simulink model "WFXXPIDzlsa"  (Simulink 5.0)
settings: Solver=ode4  SolverMode=SingleTasking  StartTime=0.0  StopTime=8000  FixedStep=10  RelTol=1e-3
settings Model: LastModifiedBy=ThinkPad

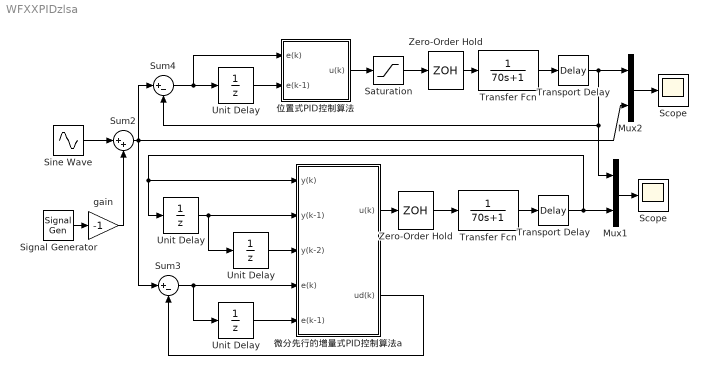
== system WFXXPIDzlsa ==
  " Unit Delay " : UnitDelay  SampleTime=20
  Mux1 : Mux  Inputs=2
  Mux2 : Mux  Inputs=2
  Saturation : Saturate  UpperLimit=10  LowerLimit=-10
  Scope : Scope
      settings: YMin=-1.5  YMax=1.5  SaveName=Scope10  DataFormat=Array  MaxDataPoints=500000
  "Scope " : Scope
      settings: YMin=-3.5  YMax=1  SaveName=ScopeData3  MaxDataPoints=500000
  Signal Generator : SignalGenerator  WaveForm=square  Frequency=0.0005*pi  Units=rad/sec
  Sine Wave : Sin  Amplitude=0.05  Frequency=0.03*pi  SampleTime=0
  Sum2 : Sum  Inputs=|++  SaturateOnIntegerOverflow=on
  Sum3 : Sum  Inputs=|+-  SaturateOnIntegerOverflow=on
  Sum4 : Sum  Inputs=|+-  SaturateOnIntegerOverflow=on
  Transfer Fcn : TransferFcn  Denominator=[70 1]
  "Transfer Fcn " : TransferFcn  Denominator=[70 1]
  Transport Delay : TransportDelay  DelayTime=80
  "Transport Delay " : TransportDelay  DelayTime=80
  Unit Delay : UnitDelay  SampleTime=20
  "Unit Delay " : UnitDelay  SampleTime=20
  "Unit Delay  " : UnitDelay  SampleTime=20
  Zero-Order Hold : ZeroOrderHold  SampleTime=20
  "Zero-Order Hold " : ZeroOrderHold  SampleTime=20
  gain : Gain  Gain=-1  SaturateOnIntegerOverflow=on
  微分先行的增量式PID控制算法a : Subsystem
  "位置式PID控制算法 " : Subsystem
  wires:
  Sum2/1 -> Sum4/1, Mux2/2, Sum3/1
  Transfer Fcn/1 -> Transport Delay/1
  "位置式PID控制算法 "/1(u(k)) -> Saturation/1
  Sum4/1 -> Unit Delay/1, "位置式PID控制算法 "/1(e(k))
  Zero-Order Hold/1 -> Transfer Fcn/1
  Mux2/1 -> Scope/1
  Transport Delay/1 -> Mux2/1, Sum4/2, Mux1/1
  Unit Delay/1 -> "位置式PID控制算法 "/2(e(k-1))
  Sine Wave/1 -> Sum2/1
  Signal Generator/1 -> gain/1
  gain/1 -> Sum2/2
  Saturation/1 -> Zero-Order Hold/1
  Sum3/1 -> 微分先行的增量式PID控制算法a/4(e(k)), "Unit Delay  "/1
  Mux1/1 -> "Scope "/1
  "Transport Delay "/1 -> "Unit Delay "/1, 微分先行的增量式PID控制算法a/1(y(k)), Mux1/2
  微分先行的增量式PID控制算法a/1(u(k)) -> "Zero-Order Hold "/1
  "Unit Delay "/1 -> " Unit Delay "/1, 微分先行的增量式PID控制算法a/2(y(k-1))
  "Unit Delay  "/1 -> 微分先行的增量式PID控制算法a/5(e(k-1))
  " Unit Delay "/1 -> 微分先行的增量式PID控制算法a/3(y(k-2))
  "Transfer Fcn "/1 -> "Transport Delay "/1
  "Zero-Order Hold "/1 -> "Transfer Fcn "/1
  微分先行的增量式PID控制算法a/2(ud(k)) -> Sum3/2

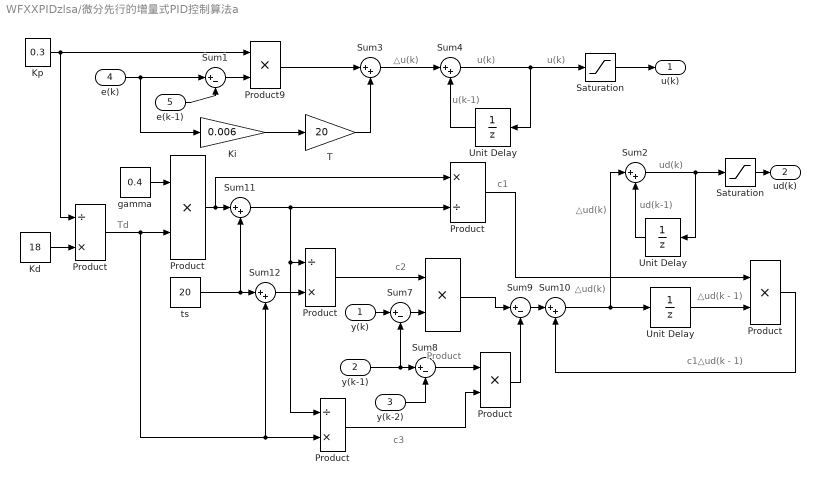
== system WFXXPIDzlsa/微分先行的增量式PID控制算法a ==
  note: u(k-1)
  note: △u(k)
  note: u(k)
  note: c1△ud(k－1)
  note: Td
  note: c2
  note: c3
  note: c1
  note: u(k)
  note: △ud(k－1)
  note: △ud(k)
  note: ud(k-1)
  note: △ud(k)
  note: ud(k)
  note: Product
  y(k) : Inport
  y(k-1) : Inport  Port=2
  y(k-2) : Inport  Port=3
  e(k) : Inport  Port=4
  e(k-1) : Inport  Port=5
  " " : Product  SaturateOnIntegerOverflow=on
  "   Product " : Product  SaturateOnIntegerOverflow=on
  "  Product " : Product  Inputs=/*  SaturateOnIntegerOverflow=on
  "  Product  " : Product  Inputs=/*  SaturateOnIntegerOverflow=on
  "  Product   " : Product  Inputs=/*  SaturateOnIntegerOverflow=on
  " Product " : Product  Inputs=*/  SaturateOnIntegerOverflow=on
  Kd : Constant  Value=18
  Ki : Gain  Gain=0.006  SaturateOnIntegerOverflow=on
  Kp : Constant  Value=0.3
  Product : Product  SaturateOnIntegerOverflow=on
  "Product  " : Product  SaturateOnIntegerOverflow=on
  Product9 : Product  SaturateOnIntegerOverflow=on
  Saturation : Saturate  UpperLimit=10  LowerLimit=-10
  "Saturation " : Saturate  UpperLimit=10  LowerLimit=-10
  Sum{1,7..9} (4 alike) : Sum  Inputs=|+-  SaturateOnIntegerOverflow=on
  Sum{2..4,10..12} (6 alike) : Sum  Inputs=|++  SaturateOnIntegerOverflow=on
  T : Gain  Gain=20  SaturateOnIntegerOverflow=on
  Unit Delay : UnitDelay  Orientation=left  SampleTime=20
  "Unit Delay " : UnitDelay  SampleTime=20
  "Unit Delay  " : UnitDelay  Orientation=left  SampleTime=20
  gamma : Constant  Value=0.4
  ts : Constant  Value=20
  u(k) : Outport
  ud(k) : Outport  Port=2
  wires:
  Product9/1 -> Sum3/1
  Ki/1 -> T/1
  Sum4/1 -> Unit Delay/1, Saturation/1
  Unit Delay/1 -> Sum4/2
  e(k-1)/1 -> Sum1/2
  Sum3/1 -> Sum4/1
  Product/1 -> Sum10/2
  Sum9/1 -> Sum10/1
  Sum10/1 -> "Unit Delay "/1, Sum2/1
  Kp/1 -> "  Product   "/1, Product9/1
  Kd/1 -> "  Product   "/2
  "Product  "/1 -> Sum11/1, " Product "/1
  ts/1 -> Sum11/2, Sum12/1
  Sum11/1 -> " Product "/2, "  Product "/1, "  Product  "/1
  "  Product   "/1 -> "Product  "/2, Sum12/2, "  Product "/2
  gamma/1 -> "Product  "/1
  Sum12/1 -> "  Product  "/2
  "  Product  "/1 -> " "/1
  "  Product "/1 -> "   Product "/2
  Sum7/1 -> " "/2
  " "/1 -> Sum9/1
  "   Product "/1 -> Sum9/2
  " Product "/1 -> Product/1
  e(k)/1 -> Sum1/1, Ki/1
  Sum1/1 -> Product9/2
  y(k)/1 -> Sum7/1
  y(k-1)/1 -> Sum7/2, Sum8/1
  y(k-2)/1 -> Sum8/2
  Sum8/1 -> "   Product "/1
  Saturation/1 -> u(k)/1
  T/1 -> Sum3/2
  "Unit Delay "/1 -> Product/2
  Sum2/1 -> "Saturation "/1, "Unit Delay  "/1
  "Unit Delay  "/1 -> Sum2/2
  "Saturation "/1 -> ud(k)/1

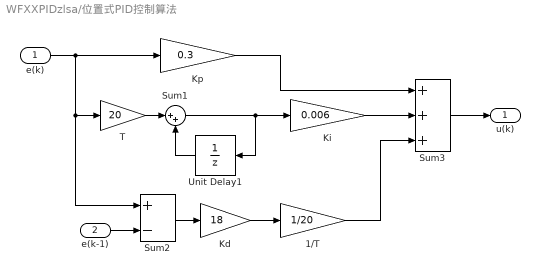
== system WFXXPIDzlsa/位置式PID控制算法  ==
  e(k) : Inport
  e(k-1) : Inport  Port=2
  1/T : Gain  Gain=1/20  SaturateOnIntegerOverflow=on
  Kd : Gain  Gain=18  SaturateOnIntegerOverflow=on
  Ki : Gain  Gain=0.006  SaturateOnIntegerOverflow=on
  Kp : Gain  Gain=0.3  SaturateOnIntegerOverflow=on
  Sum1 : Sum  Inputs=|++  SaturateOnIntegerOverflow=on
  Sum2 : Sum  Inputs=+-  SaturateOnIntegerOverflow=on
  Sum3 : Sum  Inputs=+++  SaturateOnIntegerOverflow=on
  T : Gain  Gain=20  SaturateOnIntegerOverflow=on
  Unit Delay1 : UnitDelay  Orientation=left  SampleTime=20
  u(k) : Outport
  wires:
  Sum2/1 -> Kd/1
  e(k)/1 -> Kp/1, Sum2/1, T/1
  Kp/1 -> Sum3/1
  Ki/1 -> Sum3/2
  Sum3/1 -> u(k)/1
  Kd/1 -> 1/T/1
  e(k-1)/1 -> Sum2/2
  1/T/1 -> Sum3/3
  Sum1/1 -> Unit Delay1/1, Ki/1
  Unit Delay1/1 -> Sum1/2
  T/1 -> Sum1/1
